simulink model "ClosedLoop"  (R2024a)
settings: Solver=ode4  StartTime=0.0  StopTime=30  FixedStep=DT  MaxStep=DT  RelTol=1e-3  EnableMultiTasking=on
undefined symbols (not defined in the file or in its folder): OutList, rpm2rads, strmatch
settings Model: Creator=bjonkman  LastModifiedBy=glazzerini
settings SolverCC: AlgebraicLoopSolver=TrustRegion
settings DataIOCC: LimitDataPoints=on  SaveFormat=Array  SignalLoggingSaveFormat=ModelDataLogs  SaveOutput=off  SaveTime=off  ReturnWorkspaceOutputs=off  SignalLoggingName=sigsOut
settings OptimizationCC: ExpressionDepthLimit=2147483647  LifeSpan=inf
settings DebuggingCC: SaveWithParameterizedLinksMsg=none  UnderspecifiedInitializationDetection=Classic  MergeDetectMultiDrivingBlocksExec=none  SignalResolutionControl=TryResolveAllWithWarning  MultiTaskDSMMsg=warning  MultiTaskCondExecSysMsg=none  FcnCallInpInsideContextMsg=warning  UnconnectedInputMsg=warning  UnconnectedOutputMsg=warning  UnconnectedLineMsg=warning  StateNameClashWarn=warning  SFUnexpectedBacktrackingDiag=warning  SFNoUnconditionalDefaultTransitionDiag=warning  SFExecutionAtInitializationDiag=none  ArithmeticOperatorsInVariantConditions=warning
settings HardwareCC: ProdBitPerPointer=32  ProdBitPerSizeT=32  ProdBitPerPtrDiffT=32  ProdLargestAtomicFloat=None  ProdIntDivRoundTo=Undefined  ProdEndianess=Unspecified  ProdWordSize=32  ProdHWDeviceType=32-bit Generic  TargetUnknown=on
settings ModelReferenceCC: EnableRefExpFcnMdlSchedulingChecks=on  PropagateSignalLabelsOutOfModel=off
settings SFSimCC: SimUseLocalCustomCode=off  CustomCodeUndefinedFunction=UseInterfaceOnly
settings RTWCC: RTWUseLocalCustomCode=off  GPUComputeCapability=3.5  DLArmComputeVersion=19.05
settings CodeAppCC: StateflowObjectComments=on
settings GRTTargetCC: TargetLangStandard=C89/C90 (ANSI)  CombineOutputUpdateFcns=off  GRTInterface=on
settings ConfigComp: CovMetricSettings=dw  CovSaveCumulativeToWorkspaceVar=on  CovSaveSingleToWorkspaceVar=on  CovExternalEMLEnable=off

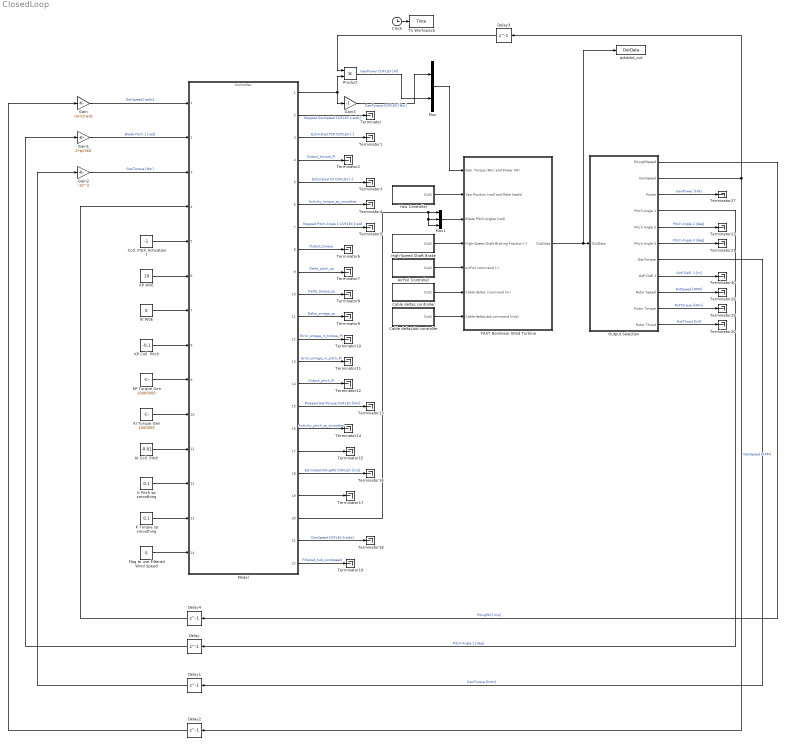
== system ClosedLoop ==
  AirFoil Controller : Subsystem
  Cable deltaL controller : Subsystem
  Cable deltaLdot controller : Subsystem
  Clock : Clock
  Coll. Pitch Activation t : Constant  Value=-1
  Delay{,1..4} (5 alike) : Delay  DelayLength=1
  FAST Nonlinear Wind Turbine : Subsystem  mask(FAST Nonlinear Wind Turbine){}
      mask help: This block contains the FAST S-Function.
      mask init:
      | clear FAST_SFunc
  Flag to use Filtered Wind Speed : Constant  Value=0
  Gain : Gain  Gain=rpm2rads
  Gain1 : Gain  Gain=2*pi/360
  Gain2 : Gain  Gain=-10^3
  Gain3 : Gain  Gain=-1
  High-Speed Shaft Brake : Subsystem
  "K Pitch sp smoothing " : Constant  Value=0.1
  "K Torque sp smoothing " : Constant  Value=0.1
  KI Coll. Pitch : Constant  Value=-0.01
  KI Torque Gen : Constant  Value=1000000
  KI WSE : Constant  Value=0
  KP Coll. Pitch : Constant  Value=-0.1
  KP Torque Gen : Constant  Value=10000000
  KP WSE : Constant  Value=10
  Model : ModelReference  ModelNameDialog=Controller.slx  SimulationMode=Normal  ModelReferenceVersion=18.122
  Mux : Mux  Inputs=2
  Mux1 : Mux  Inputs=3
  Output Selection : Subsystem
  Product : Product
  Terminator{,1..22,25..27,30} (27 alike) : Terminator
  To Workspace : ToWorkspace  VariableName=Time  SampleTime=-1
  Yaw Controller : Subsystem
  qdotdot_out : ToWorkspace  VariableName=OutData  SampleTime=-1
  wires:
  Clock/1 -> To Workspace/1
  FAST Nonlinear Wind Turbine/1(OutData) -> qdotdot_out/1, Output Selection/1(OutData)
  Mux/1 -> FAST Nonlinear Wind Turbine/1(Gen. Torque (Nm) and Power (W))
  Yaw Controller/1(Out1) -> FAST Nonlinear Wind Turbine/2(Yaw Position (rad) and Rate (rad/s))
  Model/20 -> Mux1/3, Mux1/2, Mux1/1
  High-Speed Shaft Brake/1(Out1) -> FAST Nonlinear Wind Turbine/4(High-Speed Shaft Braking Fraction (-))
  AirFoil Controller/1(Out1) -> FAST Nonlinear Wind Turbine/5(AirFoil command (-))
  Cable deltaL controller/1(Out1) -> FAST Nonlinear Wind Turbine/6(Cable deltaL command (m))
  Cable deltaLdot controller/1(Out1) -> FAST Nonlinear Wind Turbine/7(Cable deltaLdot command (m/s))
  Flag to use Filtered Wind Speed/1 -> Model/14
  KI Coll. Pitch/1 -> Model/11
  KP WSE/1 -> Model/6
  Coll. Pitch Activation t/1 -> Model/5
  KI WSE/1 -> Model/7
  KI Torque Gen/1 -> Model/10
  "K Torque sp smoothing "/1 -> Model/13
  KP Torque Gen/1 -> Model/9
  KP Coll. Pitch/1 -> Model/8
  "K Pitch sp smoothing "/1 -> Model/12
  Delay2/1 -> Gain/1
  Delay1/1 -> Gain2/1
  Output Selection/4(Pitch Angle 1) -> Delay/1  "Pitch Angle 1 [deg]"
  Delay/1 -> Gain1/1
  Output Selection/7(GenTorque) -> Delay1/1  "GenTorque [kNm]"
  Model/3 -> Terminator1/1  "Estimated TSR COFLEX [-]"
  Model/2 -> Terminator/1  "Mapped GenSpeed COFLEX [rad/s]"
  Model/5 -> Terminator3/1  "Estimated CP COFLEX [-]"
  Model/13 -> Terminator11/1  "Error_omega_in_pitch_PI"
  Model/7 -> Terminator5/1  "Mapped Pitch Angle 1 COFLEX [rad]"
  Model/15 -> Terminator13/1  "Mapped GenTorque COFLEX [Nm]"
  Model/8 -> Terminator6/1  "Output_torque"
  Model/22 -> Terminator19/1  "Filtered_hub_windspeed"
  Model/14 -> Terminator12/1  "Output_pitch_PI"
  Model/19 -> Terminator17/1
  Model/21 -> Terminator18/1  "GenSpeed COFLEX [rad/s]"
  Model/4 -> Terminator2/1  "Output_torque_PI"
  Model/6 -> Terminator4/1  "Activity_torque_sp_smoother"
  Model/17 -> Terminator15/1
  Model/10 -> Terminator8/1  "Delta_torque_sp"
  Model/11 -> Terminator9/1  "Delta_omega_sp"
  Model/18 -> Terminator16/1  "Estimated RAvgWS COFLEX [m/s]"
  Model/9 -> Terminator7/1  "Delta_pitch_sp"
  Model/12 -> Terminator10/1  "Error_omega_in_torque_PI"
  Model/16 -> Terminator14/1  "Activity_pitch_sp_smoother"
  Model/1 -> Product/2, Gain3/1
  Gain/1 -> Model/1  "GenSpeed [rad/s]"
  Gain1/1 -> Model/2  "Blade Pitch 1 [rad]"
  Gain2/1 -> Model/3  "GenTorque [Nm]"
  Product/1 -> Mux/2  "GenPower COFLEX [W]"
  Delay3/1 -> Product/1
  Output Selection/2("GenSpeed ") -> Delay3/1, Delay2/1  "GenSpeed [RPM]"
  Delay4/1 -> Model/4
  Mux1/1 -> FAST Nonlinear Wind Turbine/3(Blade Pitch Angles (rad))
  Gain3/1 -> Mux/1  "GenTorque COFLEX [Nm]"
  Output Selection/8(OoP Defl 1) -> Terminator30/1  "OoP Defl. 1 [m]"
  Output Selection/9(Rotor Speed) -> Terminator26/1  "RotSpeed [RPM]"
  Output Selection/10(Rotor Torque) -> Terminator25/1  "RotTorque [kNm]"
  Output Selection/11(Rotor Thrust) -> Terminator20/1  "RotThrust [kN]"
  Output Selection/5(Pitch Angle 2) -> Terminator22/1  "Pitch Angle 2 [deg]"
  Output Selection/6(Pitch Angle 3) -> Terminator21/1  "Pitch Angle 3 [deg]"
  Output Selection/3(Power) -> Terminator27/1  "GenPower [kW]"
  Output Selection/1(RAvgWSpeed) -> Delay4/1  "RAvgWS [m/s]"

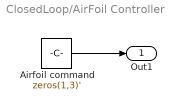
== system ClosedLoop/AirFoil Controller ==
  Airfoil command : Constant  Value=zeros(1,3)'
  Out1 : Outport
  wires:
  Airfoil command/1 -> Out1/1

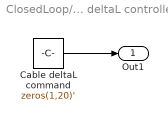
== system ClosedLoop/Cable deltaL controller ==
  Cable deltaL command : Constant  Value=zeros(1,20)'
  Out1 : Outport
  wires:
  Cable deltaL command/1 -> Out1/1

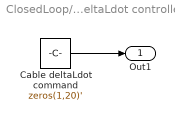
== system ClosedLoop/Cable deltaLdot controller ==
  Cable deltaLdot command : Constant  Value=zeros(1,20)'
  Out1 : Outport
  wires:
  Cable deltaLdot command/1 -> Out1/1

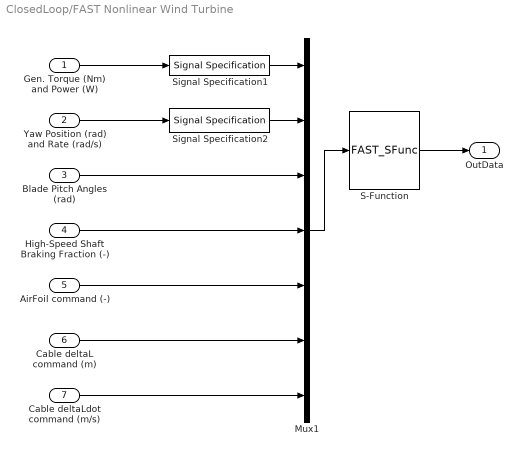
== system ClosedLoop/FAST Nonlinear Wind Turbine ==
  Gen. Torque (Nm) and Power (W) : Inport
  Yaw Position (rad) and Rate (rad/s) : Inport  Port=2
  Blade Pitch Angles (rad) : Inport  Port=3
  High-Speed Shaft Braking Fraction (-) : Inport  Port=4
  AirFoil command (-) : Inport  Port=5
  Cable deltaL command (m) : Inport  Port=6
  Cable deltaLdot command (m/s) : Inport  Port=7
  Mux1 : Mux  Inputs=7
  S-Function : S-Function  FunctionName=FAST_SFunc  Parameters=FAST_InputFileName, TMax, 0  SFunctionDeploymentMode=off  EnableBusSupport=off
  Signal Specification1 : SignalSpecification  OutDataTypeStr=double  Dimensions=2
  Signal Specification2 : SignalSpecification  OutDataTypeStr=double  Dimensions=2
  OutData : Outport
  wires:
  Gen. Torque (Nm) and Power (W)/1 -> Signal Specification1/1
  S-Function/1 -> OutData/1
  Mux1/1 -> S-Function/1
  Blade Pitch Angles (rad)/1 -> Mux1/3
  Yaw Position (rad) and Rate (rad/s)/1 -> Signal Specification2/1
  Signal Specification1/1 -> Mux1/1
  Signal Specification2/1 -> Mux1/2
  High-Speed Shaft Braking Fraction (-)/1 -> Mux1/4
  AirFoil command (-)/1 -> Mux1/5
  Cable deltaL command (m)/1 -> Mux1/6
  Cable deltaLdot command (m/s)/1 -> Mux1/7

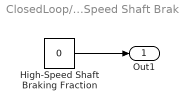
== system ClosedLoop/High-Speed Shaft Brake ==
  High-Speed Shaft Braking Fraction : Constant  Value=0
  Out1 : Outport
  wires:
  High-Speed Shaft Braking Fraction/1 -> Out1/1

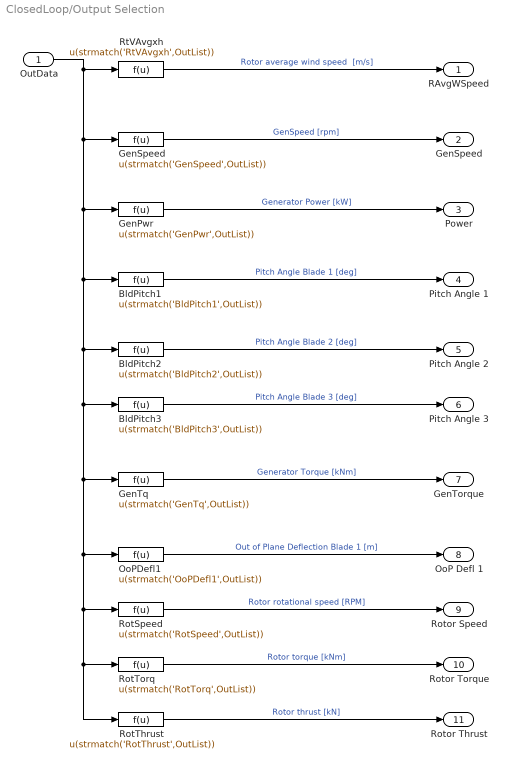
== system ClosedLoop/Output Selection ==
  OutData : Inport
  BldPitch1 : Fcn  Expr=u(strmatch('BldPitch1',OutList))
  BldPitch2 : Fcn  Expr=u(strmatch('BldPitch2',OutList))
  BldPitch3 : Fcn  Expr=u(strmatch('BldPitch3',OutList))
  GenPwr : Fcn  Expr=u(strmatch('GenPwr',OutList))
  GenSpeed : Fcn  Expr=u(strmatch('GenSpeed',OutList))
  GenTq : Fcn  Expr=u(strmatch('GenTq',OutList))
  OoPDefl1 : Fcn  Expr=u(strmatch('OoPDefl1',OutList))
  RotSpeed : Fcn  Expr=u(strmatch('RotSpeed',OutList))
  RotThrust : Fcn  Expr=u(strmatch('RotThrust',OutList))
  RotTorq : Fcn  Expr=u(strmatch('RotTorq',OutList))
  RtVAvgxh : Fcn  Expr=u(strmatch('RtVAvgxh',OutList))
  RAvgWSpeed : Outport  VectorParamsAs1DForOutWhenUnconnected=off
  "GenSpeed " : Outport  Port=2  VectorParamsAs1DForOutWhenUnconnected=off
  Power : Outport  Port=3  VectorParamsAs1DForOutWhenUnconnected=off
  Pitch Angle 1 : Outport  Port=4  VectorParamsAs1DForOutWhenUnconnected=off
  Pitch Angle 2 : Outport  Port=5  VectorParamsAs1DForOutWhenUnconnected=off
  Pitch Angle 3 : Outport  Port=6  VectorParamsAs1DForOutWhenUnconnected=off
  GenTorque : Outport  Port=7  VectorParamsAs1DForOutWhenUnconnected=off
  OoP Defl 1 : Outport  Port=8  VectorParamsAs1DForOutWhenUnconnected=off
  Rotor Speed : Outport  Port=9  VectorParamsAs1DForOutWhenUnconnected=off
  Rotor Torque : Outport  Port=10  VectorParamsAs1DForOutWhenUnconnected=off
  Rotor Thrust : Outport  Port=11  VectorParamsAs1DForOutWhenUnconnected=off
  wires:
  OutData/1 -> GenSpeed/1, GenTq/1, OoPDefl1/1, RotSpeed/1, RotTorq/1, RotThrust/1, BldPitch3/1, BldPitch2/1, BldPitch1/1, GenPwr/1, RtVAvgxh/1
  GenPwr/1 -> Power/1  "Generator Power [kW]"
  RtVAvgxh/1 -> RAvgWSpeed/1  "Rotor average wind speed  [m/s]"
  GenSpeed/1 -> "GenSpeed "/1  "GenSpeed [rpm]"
  BldPitch1/1 -> Pitch Angle 1/1  "Pitch Angle Blade 1 [deg]"
  BldPitch2/1 -> Pitch Angle 2/1  "Pitch Angle Blade 2 [deg]"
  BldPitch3/1 -> Pitch Angle 3/1  "Pitch Angle Blade 3 [deg]"
  GenTq/1 -> GenTorque/1  "Generator Torque [kNm]"
  OoPDefl1/1 -> OoP Defl 1/1  "Out of Plane Deflection Blade 1 [m]"
  RotSpeed/1 -> Rotor Speed/1  "Rotor rotational speed [RPM]"
  RotTorq/1 -> Rotor Torque/1  "Rotor torque [kNm]"
  RotThrust/1 -> Rotor Thrust/1  "Rotor thrust [kN]"

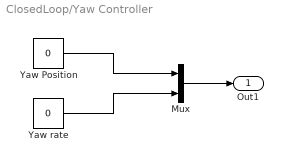
== system ClosedLoop/Yaw Controller ==
  Mux : Mux  Inputs=2
  Yaw Position : Constant  Value=0
  Yaw rate : Constant  Value=0
  Out1 : Outport
  wires:
  Mux/1 -> Out1/1
  Yaw Position/1 -> Mux/1
  Yaw rate/1 -> Mux/2
